simulink model "cw16"  (Simulink 7.0)
settings: Solver=ode4  StartTime=0.0  StopTime=10.0  FixedStep=0.01  RelTol=1e-3
values from neighbouring files (symbols this model uses):
  Beta_rate = 3*(pi/180)    (= 0.0523598775598)    [cw16set.m]
  g = 9.80665    [cw16set.m]
  gainfx = 1    [cw16set.m]
  gainfxtilt = 1    [cw16set.m]
  gainfy = 1    [cw16set.m]
  gainfytilt = 1    [cw16set.m]
  gainfz = 1    [cw16set.m]
  gainp = 1    [cw16set.m]
  gainq = 1    [cw16set.m]
  gainr = 1    [cw16set.m]
  HPomegabphi = 0.0    (= 0)    [cw16set.m]
  HPomegabpsi = 0.0    (= 0)    [cw16set.m]
  HPomegabtheta = 0.0    (= 0)    [cw16set.m]
  HPomegabx = 0.0    (= 0)    [cw16set.m]
  HPomegaby = 0.0    (= 0)    [cw16set.m]
  HPomegabz = 0.2    [cw16set.m]
  HPomeganphi = 1.0    (= 1)    [cw16set.m]
  HPomeganpsi = 1.0    (= 1)    [cw16set.m]
  HPomegantheta = 0.8    [cw16set.m]
  HPomeganx = 0.8    [cw16set.m]
  HPomegany = 1.0    (= 1)    [cw16set.m]
  HPomeganz = 1.0    (= 1)    [cw16set.m]
  HPzetaphi = 1.0    (= 1)    [cw16set.m]
  HPzetapsi = 1.0    (= 1)    [cw16set.m]
  HPzetatheta = 1.0    (= 1)    [cw16set.m]
  HPzetax = 1.0    (= 1)    [cw16set.m]
  HPzetay = 1.0    (= 1)    [cw16set.m]
  HPzetaz = 1.0    (= 1)    [cw16set.m]
  kf = [kfx 0 0; 0 kfy 0; 0 0 kfz]    [cw16set.m]
  Kfeedbackeuler = 0.2    [cw16set.m]
  Kfeedbackeulerrate = 0.5    [cw16set.m]
  Kfeedbackx = 0.5    [cw16set.m]
  Kfeedbackxd = 0.1    [cw16set.m]
  Ktilteuler = 0.2    [cw16set.m]
  Ktilteulerrate = 0.5    [cw16set.m]
  Ktiltrate = 5.0    (= 5)    [cw16set.m]
  kw = [kwp 0 0; 0 kwq 0; 0 0 kwr]    [cw16set.m]
  LPomeganx = 2.0    (= 2)    [cw16set.m]
  LPomegany = 2.0    (= 2)    [cw16set.m]
  LPzetax = 1.0    (= 1)    [cw16set.m]
  LPzetay = 1.0    (= 1)    [cw16set.m]
  LZDERPUGP = 1.2075    [cw16set.m]
  tiltcoordinationmethod = 1    [cw16set.m]
  xref_ac = 0.0    (= 0)    [cw16set.m]
  xref_filt = 0.0    (= 0)    [cw16set.m]
  yref_ac = 0.0    (= 0)    [cw16set.m]
  yref_filt = 0.0    (= 0)    [cw16set.m]
  zref_ac = -1.2075    [cw16set.m]
  zref_filt = 0.0    (= 0)    [cw16set.m]
libraries: simulink x4
(part 1 of 2)
settings Model: Creator=ostroosma  LastModifiedBy=ostroosma  ModifiedHistory=1.96: changed frequency of differentiating filters in tilt coordination from 12.5 to 50 rad/s  ParamWorkspaceSource=ReferencedWorkspace  ExtModeTrigMode=oneshot  ExtModeArmWhenConnect=off  TunableVars=Beta_rate,HPomegabphi,HPomegabpsi,HPomegabtheta,HPomegabx,HPomegaby,HPomegabz,HPomeganphi,HPomeganpsi,HPomegantheta,HPomeganx,HPomegany,HPomeganz,HPzetaphi,HPzetapsi,HPzetatheta,HPzetax,HPzetay,HPzetaz,Ktilteuler,Ktilteulerrate,Ktiltrate,LPomeganx,LPomegany,LPzetax,LPzetay,gainfx,gainfxtilt,gainfy,gainfytilt,gainfz,gainp,gainq,gainr,kf,kw,tiltcoordinationmethod,xref_ac,xref_filt,yref_ac,yref_filt,zref_ac,zref_filt  TunableVarsStorageClass=Auto,Auto,Auto,Auto,Auto,Auto,Auto,Auto,Auto,Auto,Auto,Auto,Auto,Auto,Auto,Auto,Auto,Auto,Auto,Auto,Auto,Auto,Auto,Auto,Auto,Auto,Auto,Auto,Auto,Auto,Auto,Auto,Auto,Auto,Auto,Auto,Auto,Auto,Auto,Auto,Auto,Auto,Auto  TunableVarsTypeQualifier=,,,,,,,,,,,,,,,,,,,,,,,,,,,,,,,,,,,,,,,,,,
settings DataIOCC: LimitDataPoints=off  SaveOutput=off  SignalLogging=off  SaveTime=off  SignalLoggingName=sigsOut
settings OptimizationCC: BooleanDataType=off  InlineParams=on
settings DebuggingCC: SaveWithParameterizedLinksMsg=none  SignalResolutionControl=TryResolveAllWithWarning  SolverPrmCheckMsg=none  MultiTaskDSMMsg=warning  MultiTaskCondExecSysMsg=none  FcnCallInpInsideContextMsg=Enable All  StrictBusMsg=ErrorLevel1
settings HardwareCC: TargetEndianess=LittleEndian  TargetHWDeviceType=MATLAB Host
settings RTWCC: SystemTargetFile=grt_malloc.tlc  GenCodeOnly=on  GenerateMakefile=off  TemplateMakefile=grt_malloc_default_tmf  Description=Generic Real-Time Target with dynamic memory allocation  ProcessScript=grt_malloc_make_rtw_hook  IncludeERTFirstTime=on
settings GRTTargetCC: ExtModeMexFile=noextcomm

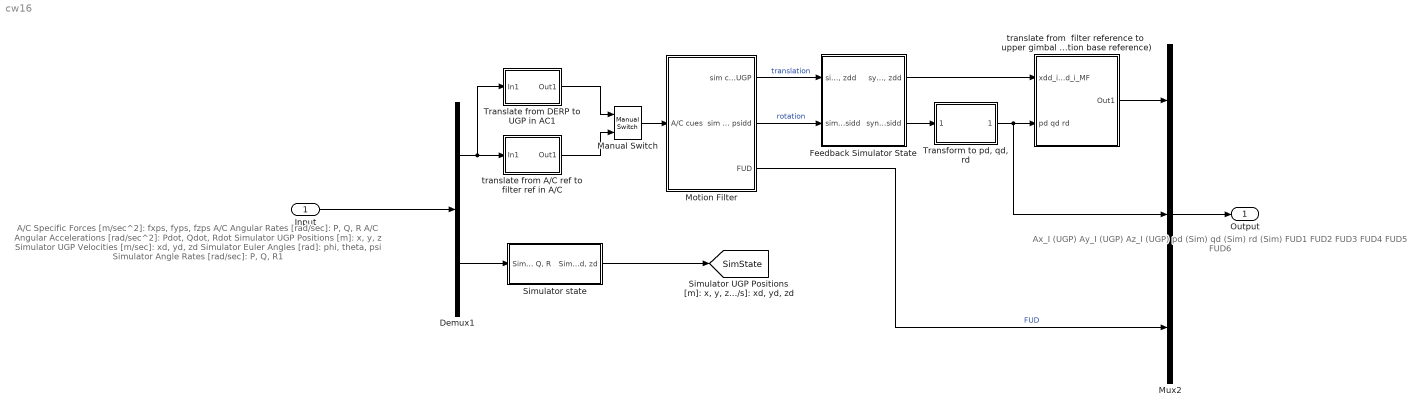
== system cw16 ==
  note: Ax_I (UGP)
      | Ay_I (UGP)
      | Az_I (UGP)
      | pd (Sim)
      | qd (Sim)
      | rd (Sim)
      | FUD1
      | FUD2
      | FUD3
      | FUD4
      | FUD5
      | FUD6
  note: A/C Specific Forces [m/sec^2]: fxps, fyps, fzps
      | A/C Angular Rates [rad/sec]: P, Q, R
      | A/C Angular Accelerations [rad/sec^2]: Pdot, Qdot, Rdot
      | Simulator UGP Positions [m]: x, y, z
      | Simulator UGP Velocities [m/sec]: xd, yd, zd
      | Simulator Euler Angles [rad]: phi, theta, psi
      | Simulator Angle Rates [rad/sec]: P, Q, R1
  Input : Inport
  Demux1 : Demux  Outputs=[9;12]
  Feedback Simulator State : Subsystem
  Manual Switch : simulink/Signal Routing/Manual Switch  SystemSampleTime=-1  sw=0  action=0  varsize=off
  Motion Filter : Subsystem
  Mux2 : Mux  Inputs=3
  Simulator state : Subsystem
  "Transform to pd, qd, rd" : Subsystem
  Translate from DERP to UGP in AC1 : Subsystem
  translate from  filter reference to  upper gimbal point  (motion base reference) : Subsystem
  translate from A/C ref to filter ref in A/C : Subsystem
  Output : Outport
  tag scope: SimState=global
  wires:
  Input/1 -> Demux1/1
  Motion Filter/1(sim commands: xdd_i_UGP ydd_i_UGP zdd_i_UGP) -> Feedback Simulator State/1("sim commands xdd, ydd, zdd")  "translation"
  Motion Filter/2(sim commands: phidd thetadd psidd) -> Feedback Simulator State/2(sim commands phidd thetadd psidd)  "rotation"
  Feedback Simulator State/2("synchronizing phidd, thetadd, psidd") -> "Transform to pd, qd, rd"/1(commands 1: phidd 2: thetadd 3: psidd)
  "Transform to pd, qd, rd"/1(pd qd rd) -> Mux2/2, translate from  filter reference to  upper gimbal point  (motion base reference)/2(pd qd rd)
  Mux2/1 -> Output/1
  Motion Filter/3(FUD) -> Mux2/3  "FUD"
  Demux1/1 -> Translate from DERP to UGP in AC1/1(In1), translate from A/C ref to filter ref in A/C/1(In1)
  Translate from DERP to UGP in AC1/1(Out1) -> Manual Switch/1
  translate from A/C ref to filter ref in A/C/1(Out1) -> Manual Switch/2
  Manual Switch/1 -> Motion Filter/1(A/C cues)
  Feedback Simulator State/1("synchronizing xdd, ydd, zdd") -> translate from  filter reference to  upper gimbal point  (motion base reference)/1(xdd_i_MF ydd_i_MF zdd_i_MF)
  translate from  filter reference to  upper gimbal point  (motion base reference)/1(Out1) -> Mux2/1
  Simulator state/1("Simulator UGP Positions [m]: x, y, z Simulator UGP Velocities [m/sec]: xd, yd, zd Simulator Euler Angles [rad]: phi, theta, psi Simulator Angle Rates [rad/sec]: P, Q, R Simulator Euler Angle Rates [rad/s]: phid, thetad, psid Simulator Filter Positions [m]: x, y, z Simulator Filter Velocities [m/s]: xd, yd, zd") -> [SimState]
  Demux1/2 -> Simulator state/1("Simulator UGP Positions [m]: x, y, z Simulator UGP Velocities [m/sec]: xd, yd, zd Simulator Euler Angles [rad]: phi, theta, psi Simulator Angle Rates [rad/sec]: P, Q, R")

== system cw16/Feedback Simulator State ==
  "sim commands xdd, ydd, zdd" : Inport
  sim commands phidd thetadd psidd : Inport  Port=2
  Demux : Demux  Outputs=[6;6]
  Euler angle and angular rate Feedback : Subsystem
  Position Velocity Feedback : Subsystem
  Sum4 : Sum  Inputs=|++  SaturateOnIntegerOverflow=on  InputSameDT=on
  Sum5 : Sum  Inputs=++|  SaturateOnIntegerOverflow=on  InputSameDT=on
  "x, y, z xd, yd, zd phi, theta, psi phid, thetad, psid" : Selector  InputPortWidth=21  IndexOptions=Index vector (dialog)  Indices=[16 17 18 19 20 21 7 8 9 13 14 15]  OutputSizes=1
  "synchronizing xdd, ydd, zdd" : Outport
  "synchronizing phidd, thetadd, psidd" : Outport  Port=2
  wires:
  sim commands phidd thetadd psidd/1 -> Sum4/1, Euler angle and angular rate Feedback/1("Simulator desired angular accelerations ")
  "sim commands xdd, ydd, zdd"/1 -> Sum5/2, Position Velocity Feedback/2("Simulator desired accelerations ")
  Euler angle and angular rate Feedback/1(feedback angular acceleration) -> Sum4/2
  Sum5/1 -> "synchronizing xdd, ydd, zdd"/1
  Sum4/1 -> "synchronizing phidd, thetadd, psidd"/1
  "x, y, z xd, yd, zd phi, theta, psi phid, thetad, psid"/1 -> Demux/1
  Demux/2 -> Euler angle and angular rate Feedback/2(feedback simulator state)
  Demux/1 -> Position Velocity Feedback/1(feedback simulator state)
  Position Velocity Feedback/1(feedback acceleration) -> Sum5/1
  [SimState] -> "x, y, z xd, yd, zd phi, theta, psi phid, thetad, psid"/1

== system cw16/Motion Filter ==
  A/C cues : Inport
  Demux1 : Demux  Outputs=[3;6]
  High Pass Channel Angular Accelerations : Subsystem
  High Pass Channel Specific Forces : Subsystem
  Low Pass Channel Specific Forces : Subsystem
  Sum1 : Sum  Inputs=++|  SaturateOnIntegerOverflow=on  InputSameDT=on
  f-scale : Subsystem
  w-scale : Subsystem
  sim commands: xdd_i_UGP ydd_i_UGP zdd_i_UGP : Outport
  sim commands: phidd thetadd psidd : Outport  Port=2
  FUD : Outport  Port=3
  wires:
  f-scale/1(scaled A/C specific force UGP) -> Low Pass Channel Specific Forces/1(scaled AC specific forces @ UGP), High Pass Channel Specific Forces/1(In1)
  Low Pass Channel Specific Forces/1(phidd LP thetadd LP psidd LP) -> Sum1/1
  Demux1/1 -> f-scale/1(A/C specific forces UGP)
  High Pass Channel Specific Forces/1(Out1) -> sim commands: xdd_i_UGP ydd_i_UGP zdd_i_UGP/1
  A/C cues/1 -> Demux1/1
  Sum1/1 -> sim commands: phidd thetadd psidd/1
  High Pass Channel Angular Accelerations/1(Out1) -> Sum1/2
  Demux1/2 -> w-scale/1(In1)
  w-scale/1(Out1) -> High Pass Channel Angular Accelerations/1(In1)
  Low Pass Channel Specific Forces/2(FUD) -> FUD/1

== system cw16/Simulator state ==
  "Simulator UGP Positions [m]: x, y, z Simulator UGP Velocities [m/sec]: xd, yd, zd Simulator Euler Angles [rad]: phi, theta, psi Simulator Angle Rates [rad/sec]: P, Q, R" : Inport
  Demux : Demux  Outputs=[6 6]
  Demux1 : Demux  Outputs=[3 3]
  Mux : Mux  Inputs=[6 6 3 3 3]
  "calculate position and velocity in filter reference point, for state feedback inside filter" : Stateflow chart  TreatAsAtomicUnit=on
  phi_s theta_s psi_s p_s q_s r_s : Selector  InputPortWidth=12  IndexOptions=Index vector (dialog)  Indices=[7 8 9 10 11 12]  OutputSizes=1
  reference points : Subsystem
  transformation to Euler angle rates : Subsystem
  "Simulator UGP Positions [m]: x, y, z Simulator UGP Velocities [m/sec]: xd, yd, zd Simulator Euler Angles [rad]: phi, theta, psi Simulator Angle Rates [rad/sec]: P, Q, R Simulator Euler Angle Rates [rad/s]: phid, thetad, psid Simulator Filter Positions [m]: x, y, z Simulator Filter Velocities [m/s]: xd, yd, zd" : Outport
  wires:
  "Simulator UGP Positions [m]: x, y, z Simulator UGP Velocities [m/sec]: xd, yd, zd Simulator Euler Angles [rad]: phi, theta, psi Simulator Angle Rates [rad/sec]: P, Q, R"/1 -> phi_s theta_s psi_s p_s q_s r_s/1, Demux/1
  Mux/1 -> "Simulator UGP Positions [m]: x, y, z Simulator UGP Velocities [m/sec]: xd, yd, zd Simulator Euler Angles [rad]: phi, theta, psi Simulator Angle Rates [rad/sec]: P, Q, R Simulator Euler Angle Rates [rad/s]: phid, thetad, psid Simulator Filter Positions [m]: x, y, z Simulator Filter Velocities [m/s]: xd, yd, zd"/1
  Demux/1 -> Demux1/1, Mux/1
  Demux/2 -> Mux/2, transformation to Euler angle rates/1("phi theta psi p q r ")
  transformation to Euler angle rates/1(phidot thetadot psidot) -> Mux/3
  reference points/1(Out1) -> "calculate position and velocity in filter reference point, for state feedback inside filter"/4(refpos)
  phi_s theta_s psi_s p_s q_s r_s/1 -> "calculate position and velocity in filter reference point, for state feedback inside filter"/3(attsim)
  Demux1/2 -> "calculate position and velocity in filter reference point, for state feedback inside filter"/2(xd_ugp)
  Demux1/1 -> "calculate position and velocity in filter reference point, for state feedback inside filter"/1(x_ugp)
  "calculate position and velocity in filter reference point, for state feedback inside filter"/1(x_filt) -> Mux/4
  "calculate position and velocity in filter reference point, for state feedback inside filter"/2(xd_filt) -> Mux/5

== system cw16/Transform to pd, qd, rd ==
  note: differentiated formula 2.14 from UTIAS
  note: WHY, it's in SimState already?
  commands 1: phidd 2: thetadd 3: psidd : Inport
  7: phi 8: theta 9: psi 10: phid 11: thetad 12: psid : Selector  InputPortWidth=21  IndexOptions=Index vector (dialog)  Indices=[7 8 9 13 14 15]  OutputSizes=1
  Integrate to  4: phid 5: thetad 6: psid : Subsystem
  Mux : Mux  Inputs=3
  Mux1 : Mux  Inputs=3
  pd : Fcn  Expr=-cos(u[8])*u[11]*u[6]+u[1]-sin(u[8])*u[3]
  qd : Fcn  Expr=-sin(u[7])*u[10]*u[5]+(cos(u[8])*cos(u[7])*u[10]-sin(u[8])*u[11]*sin(u[7]))*u[6]+cos(u[7])*u[2]+cos(u[8])*sin(u[7])*u[3]
  rd : Fcn  Expr=-cos(u[7])*u[10]*u[5]-(sin(u[8])*u[11]*cos(u[7])+cos(u[8])*sin(u[7])*u[10])*u[6]-sin(u[7])*u[2]+cos(u[8])*cos(u[7])*u[3]
  pd qd rd : Outport
  wires:
  commands 1: phidd 2: thetadd 3: psidd/1 -> Integrate to  4: phid 5: thetad 6: psid/1(In1), Mux/1
  Integrate to  4: phid 5: thetad 6: psid/1(Out1) -> Mux/2
  Mux/1 -> pd/1, qd/1, rd/1
  qd/1 -> Mux1/2
  rd/1 -> Mux1/3
  pd/1 -> Mux1/1
  Mux1/1 -> pd qd rd/1
  [SimState] -> 7: phi 8: theta 9: psi 10: phid 11: thetad 12: psid/1
  7: phi 8: theta 9: psi 10: phid 11: thetad 12: psid/1 -> Mux/3

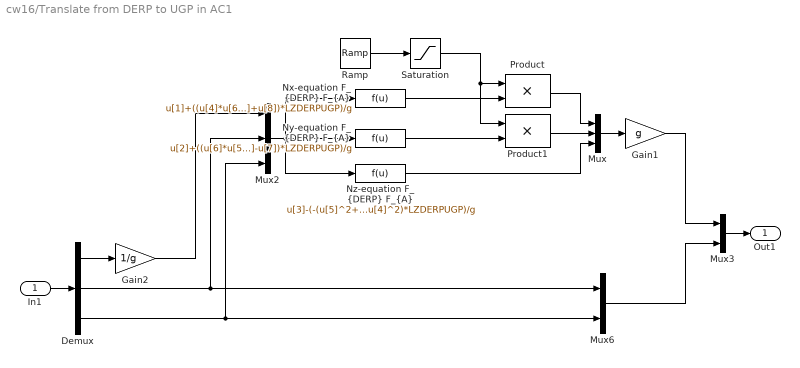
== system cw16/Translate from DERP to UGP in AC1 ==
  In1 : Inport
  Demux : Demux  Outputs=[3;3;3]
  Gain1 : Gain  Gain=g  SaturateOnIntegerOverflow=on
  Gain2 : Gain  Gain=1/g  SaturateOnIntegerOverflow=on
  Mux : Mux  Inputs=3
  Mux2 : Mux  Inputs=3
  Mux3 : Mux  Inputs=2
  Mux6 : Mux  Inputs=2
  "Nx-equation F_{DERP} F_{A}" : Fcn  Expr=u[1]+((u[4]*u[6]+u[8])*LZDERPUGP)/g
  "Ny-equation F_{DERP} F_{A}" : Fcn  Expr=u[2]+((u[6]*u[5]-u[7])*LZDERPUGP)/g
  "Nz-equation F_{DERP} F_{A}" : Fcn  Expr=u[3]-(-(u[5]^2+u[4]^2)*LZDERPUGP)/g
  Product : Product  SaturateOnIntegerOverflow=on  InputSameDT=on
  Product1 : Product  SaturateOnIntegerOverflow=on  InputSameDT=on
  Ramp : simulink/Sources/Ramp  SystemSampleTime=-1  slope=0.2  start=0  X0=0
  Saturation : Saturate  UpperLimit=1  LowerLimit=0
  Out1 : Outport
  wires:
  Mux2/1 -> "Ny-equation F_{DERP} F_{A}"/1, "Nx-equation F_{DERP} F_{A}"/1, "Nz-equation F_{DERP} F_{A}"/1
  Ramp/1 -> Saturation/1
  Mux/1 -> Gain1/1
  Product/1 -> Mux/1
  "Nx-equation F_{DERP} F_{A}"/1 -> Product/2
  Product1/1 -> Mux/2
  "Ny-equation F_{DERP} F_{A}"/1 -> Product1/2
  Saturation/1 -> Product/1, Product1/1
  Gain1/1 -> Mux3/1
  Mux6/1 -> Mux3/2
  Mux3/1 -> Out1/1
  In1/1 -> Demux/1
  Demux/3 -> Mux2/3, Mux6/2
  Demux/2 -> Mux2/2, Mux6/1
  Demux/1 -> Gain2/1
  Gain2/1 -> Mux2/1
  "Nz-equation F_{DERP} F_{A}"/1 -> Mux/3

== system cw16/translate from  filter reference to  upper gimbal point  (motion base reference) ==
  xdd_i_MF ydd_i_MF zdd_i_MF : Inport  PortDimensions=3
  pd qd rd : Inport  Port=2
  move inertial acceleration setpoints in MF reference point to UGP reference point : Stateflow chart  TreatAsAtomicUnit=on
  phi_s theta_s psi_s p_s q_s r_s : Selector  InputPortWidth=21  IndexOptions=Index vector (dialog)  Indices=[7 8 9 10 11 12]  OutputSizes=1
  reference points : Subsystem
  Out1 : Outport
  wires:
  xdd_i_MF ydd_i_MF zdd_i_MF/1 -> move inertial acceleration setpoints in MF reference point to UGP reference point/1(xdd_i_mf)
  reference points/1(Out1) -> move inertial acceleration setpoints in MF reference point to UGP reference point/4(refpos)
  move inertial acceleration setpoints in MF reference point to UGP reference point/1(xdd_i_ugp) -> Out1/1
  pd qd rd/1 -> move inertial acceleration setpoints in MF reference point to UGP reference point/2(wd_mf)
  [SimState] -> phi_s theta_s psi_s p_s q_s r_s/1
  phi_s theta_s psi_s p_s q_s r_s/1 -> move inertial acceleration setpoints in MF reference point to UGP reference point/3(attsim)

== system cw16/translate from A/C ref to filter ref in A/C ==
  note: fade in fx/fy
  In1 : Inport
  Demux : Demux  Outputs=[2 7]
  Embedded MATLAB Function : Stateflow chart  TreatAsAtomicUnit=on
  Mux : Mux  Inputs=[2 7]
  Product : Product  SaturateOnIntegerOverflow=on  InputSameDT=on
  Ramp : simulink/Sources/Ramp  SystemSampleTime=-1  slope=0.2  start=0  X0=0
  Saturation : Saturate  UpperLimit=1  LowerLimit=0
  reference points : Subsystem
  Out1 : Outport
  wires:
  Embedded MATLAB Function/1(y) -> Out1/1
  reference points/1(Out1) -> Embedded MATLAB Function/2(refpos)
  Ramp/1 -> Saturation/1
  Saturation/1 -> Product/1
  In1/1 -> Demux/1
  Demux/1 -> Product/2
  Product/1 -> Mux/1
  Demux/2 -> Mux/2
  Mux/1 -> Embedded MATLAB Function/1(u)

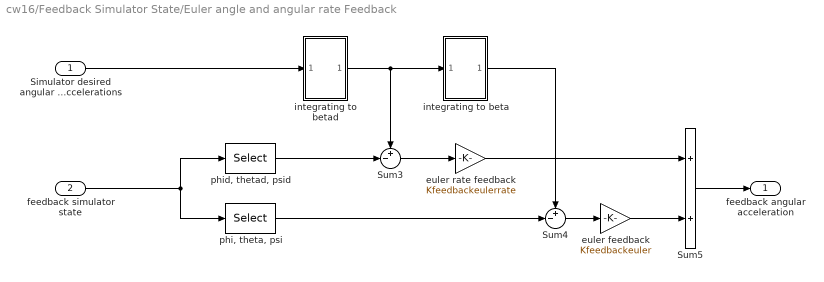
== system cw16/Feedback Simulator State/Euler angle and angular rate Feedback ==
  "Simulator desired angular accelerations " : Inport
  feedback simulator state : Inport  Port=2
  Sum3 : Sum  Inputs=+-|  SaturateOnIntegerOverflow=on  InputSameDT=on
  Sum4 : Sum  Inputs=+-|  SaturateOnIntegerOverflow=on  InputSameDT=on
  Sum5 : Sum  SaturateOnIntegerOverflow=on  InputSameDT=on
  euler feedback : Gain  Gain=Kfeedbackeuler  SaturateOnIntegerOverflow=on
  euler rate feedback : Gain  Gain=Kfeedbackeulerrate  SaturateOnIntegerOverflow=on
  integrating to beta : Subsystem
  integrating to betad : Subsystem
  "phi, theta, psi" : Selector  InputPortWidth=6  IndexOptions=Index vector (dialog)  Indices=[1 2 3]  OutputSizes=1
  "phid, thetad, psid" : Selector  InputPortWidth=6  IndexOptions=Index vector (dialog)  Indices=[4 5 6]  OutputSizes=1
  feedback angular acceleration : Outport
  wires:
  "Simulator desired angular accelerations "/1 -> integrating to betad/1(In1)
  integrating to betad/1(Out1) -> integrating to beta/1(In1), Sum3/1
  Sum3/1 -> euler rate feedback/1
  feedback simulator state/1 -> "phi, theta, psi"/1, "phid, thetad, psid"/1
  integrating to beta/1(Out1) -> Sum4/1
  Sum4/1 -> euler feedback/1
  euler feedback/1 -> Sum5/2
  euler rate feedback/1 -> Sum5/1
  Sum5/1 -> feedback angular acceleration/1
  "phi, theta, psi"/1 -> Sum4/2
  "phid, thetad, psid"/1 -> Sum3/2

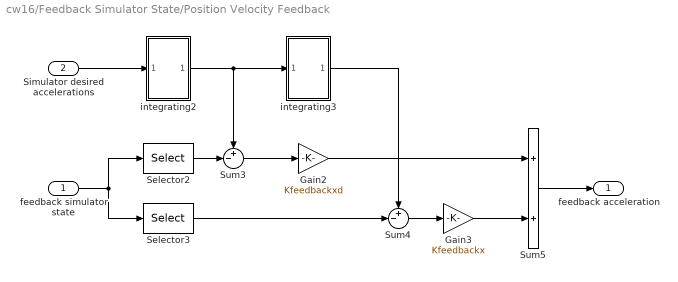
== system cw16/Feedback Simulator State/Position Velocity Feedback ==
  feedback simulator state : Inport
  "Simulator desired accelerations " : Inport  Port=2
  Gain2 : Gain  Gain=Kfeedbackxd  SaturateOnIntegerOverflow=on
  Gain3 : Gain  Gain=Kfeedbackx  SaturateOnIntegerOverflow=on
  Selector2 : Selector  InputPortWidth=6  IndexOptions=Index vector (dialog)  Indices=[4 5 6]  OutputSizes=1
  Selector3 : Selector  InputPortWidth=6  IndexOptions=Index vector (dialog)  Indices=[1 2 3]  OutputSizes=1
  Sum3 : Sum  Inputs=+-|  SaturateOnIntegerOverflow=on  InputSameDT=on
  Sum4 : Sum  Inputs=+-|  SaturateOnIntegerOverflow=on  InputSameDT=on
  Sum5 : Sum  SaturateOnIntegerOverflow=on  InputSameDT=on
  integrating2 : Subsystem
  integrating3 : Subsystem
  feedback acceleration : Outport
  wires:
  "Simulator desired accelerations "/1 -> integrating2/1(In1)
  Selector2/1 -> Sum3/2
  integrating2/1(Out1) -> integrating3/1(In1), Sum3/1
  Sum3/1 -> Gain2/1
  feedback simulator state/1 -> Selector2/1, Selector3/1
  Selector3/1 -> Sum4/2
  integrating3/1(Out1) -> Sum4/1
  Sum4/1 -> Gain3/1
  Gain3/1 -> Sum5/2
  Gain2/1 -> Sum5/1
  Sum5/1 -> feedback acceleration/1

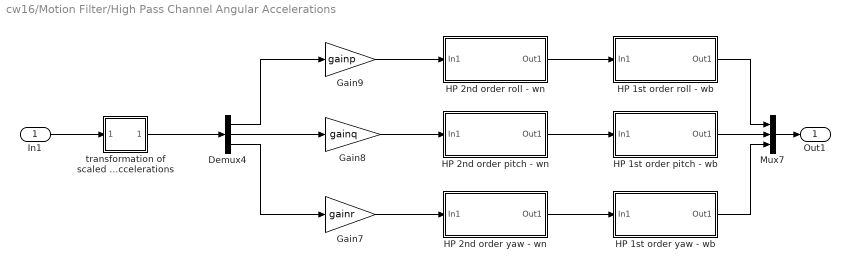
== system cw16/Motion Filter/High Pass Channel Angular Accelerations ==
  In1 : Inport
  Demux4 : Demux  Outputs=3
  Gain7 : Gain  Gain=gainr  SaturateOnIntegerOverflow=on
  Gain8 : Gain  Gain=gainq  SaturateOnIntegerOverflow=on
  Gain9 : Gain  Gain=gainp  SaturateOnIntegerOverflow=on
  HP 1st order pitch - wb : Subsystem
  HP 1st order roll - wb : Subsystem
  HP 1st order yaw - wb : Subsystem
  HP 2nd order pitch - wn : Subsystem
  HP 2nd order roll - wn : Subsystem
  HP 2nd order yaw - wn : Subsystem
  Mux7 : Mux  Inputs=3
  transformation of scaled A/C rotations to sim Euler angle accelerations : Subsystem
  Out1 : Outport
  wires:
  Gain7/1 -> HP 2nd order yaw - wn/1(In1)
  Gain8/1 -> HP 2nd order pitch - wn/1(In1)
  Gain9/1 -> HP 2nd order roll - wn/1(In1)
  Demux4/1 -> Gain9/1
  Demux4/3 -> Gain7/1
  In1/1 -> transformation of scaled A/C rotations to sim Euler angle accelerations/1(1: p (A/C) 2: q (A/C) 3: r (A/C) 4: pd (A/C) 5: qd (A/C) 6: rd (A/C))
  Demux4/2 -> Gain8/1
  transformation of scaled A/C rotations to sim Euler angle accelerations/1(phidd thetadd psidd) -> Demux4/1
  Mux7/1 -> Out1/1
  HP 1st order roll - wb/1(Out1) -> Mux7/1
  HP 1st order pitch - wb/1(Out1) -> Mux7/2
  HP 1st order yaw - wb/1(Out1) -> Mux7/3
  HP 2nd order roll - wn/1(Out1) -> HP 1st order roll - wb/1(In1)
  HP 2nd order pitch - wn/1(Out1) -> HP 1st order pitch - wb/1(In1)
  HP 2nd order yaw - wn/1(Out1) -> HP 1st order yaw - wb/1(In1)

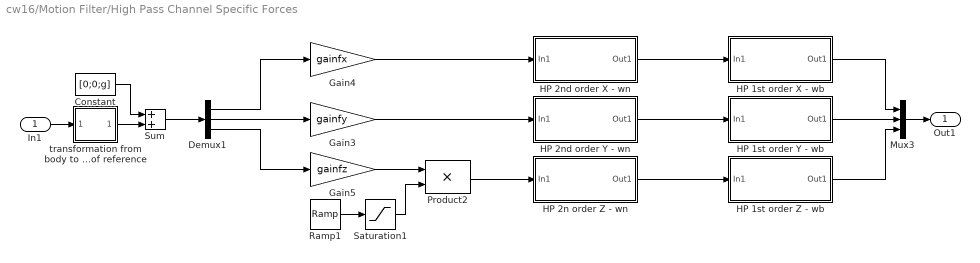
== system cw16/Motion Filter/High Pass Channel Specific Forces ==
  In1 : Inport
  Constant : Constant  Value=[0;0;g]
  Demux1 : Demux  Outputs=3
  Gain3 : Gain  Gain=gainfy  SaturateOnIntegerOverflow=on
  Gain4 : Gain  Gain=gainfx  SaturateOnIntegerOverflow=on
  Gain5 : Gain  Gain=gainfz  SaturateOnIntegerOverflow=on
  HP 1st order X - wb : Subsystem
  HP 1st order Y - wb : Subsystem
  HP 1st order Z - wb : Subsystem
  HP 2n order Z - wn : Subsystem
  HP 2nd order X - wn : Subsystem
  HP 2nd order Y - wn : Subsystem
  Mux3 : Mux  Inputs=3
  Product2 : Product  SaturateOnIntegerOverflow=on  InputSameDT=on
  Ramp1 : simulink/Sources/Ramp  SystemSampleTime=-1  slope=0.2  start=0  X0=0
  Saturation1 : Saturate  UpperLimit=1  LowerLimit=0
  Sum : Sum  SaturateOnIntegerOverflow=on  InputSameDT=on
  transformation from body to inertial frame of reference : Subsystem
  Out1 : Outport
  wires:
  transformation from body to inertial frame of reference/1(fxI fyI fzI) -> Sum/2
  Constant/1 -> Sum/1
  Sum/1 -> Demux1/1
  Demux1/2 -> Gain3/1
  Demux1/1 -> Gain4/1
  Demux1/3 -> Gain5/1
  Gain3/1 -> HP 2nd order Y - wn/1(In1)
  HP 2nd order Y - wn/1(Out1) -> HP 1st order Y - wb/1(In1)
  HP 2nd order X - wn/1(Out1) -> HP 1st order X - wb/1(In1)
  HP 2n order Z - wn/1(Out1) -> HP 1st order Z - wb/1(In1)
  HP 1st order Y - wb/1(Out1) -> Mux3/2
  Product2/1 -> HP 2n order Z - wn/1(In1)
  Gain5/1 -> Product2/1
  Saturation1/1 -> Product2/2
  Ramp1/1 -> Saturation1/1
  HP 1st order Z - wb/1(Out1) -> Mux3/3
  Mux3/1 -> Out1/1
  In1/1 -> transformation from body to inertial frame of reference/1(fxS fyS fzS)
  HP 1st order X - wb/1(Out1) -> Mux3/1
  Gain4/1 -> HP 2nd order X - wn/1(In1)

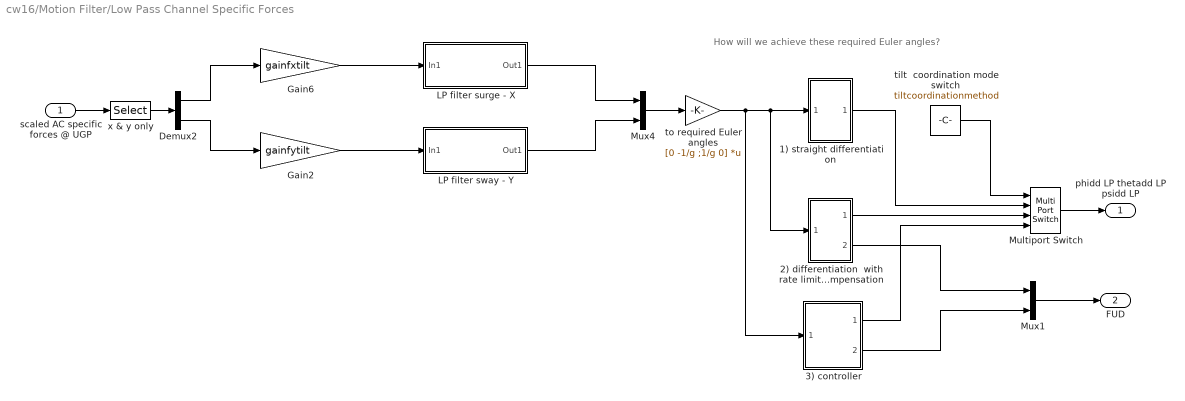
== system cw16/Motion Filter/Low Pass Channel Specific Forces ==
  note: How will we achieve
      | these required Euler angles?
  scaled AC specific forces @ UGP : Inport
  1) straight differentiation : Subsystem
  2) differentiation  with rate limit  compensation : Subsystem
  3) controller : Subsystem
  Demux2 : Demux  Outputs=2
  Gain2 : Gain  Gain=gainfytilt  SaturateOnIntegerOverflow=on
  Gain6 : Gain  Gain=gainfxtilt  SaturateOnIntegerOverflow=on
  "LP filter surge - X " : Subsystem
  "LP filter sway - Y " : Subsystem
  Multiport Switch : MultiPortSwitch  Inputs=3  SaturateOnIntegerOverflow=on
  Mux1 : Mux  Inputs=[3 3]
  Mux4 : Mux  Inputs=2
  tilt  coordination mode switch : Constant  Value=tiltcoordinationmethod
  to required Euler angles : Gain  Gain=[0 -1/g ;1/g 0]  Multiplication=Matrix(K*u)  SaturateOnIntegerOverflow=on
  x & y only : Selector  InputPortWidth=3  IndexOptions=Index vector (dialog)  Indices=[1 2]  OutputSizes=1
  phidd LP thetadd LP psidd LP : Outport
  FUD : Outport  Port=2
  wires:
  scaled AC specific forces @ UGP/1 -> x & y only/1
  x & y only/1 -> Demux2/1
  Gain2/1 -> "LP filter sway - Y "/1(In1)
  Gain6/1 -> "LP filter surge - X "/1(In1)
  "LP filter sway - Y "/1(Out1) -> Mux4/2
  "LP filter surge - X "/1(Out1) -> Mux4/1
  Mux4/1 -> to required Euler angles/1
  to required Euler angles/1 -> 3) controller/1(required Euler angles: phi theta), 1) straight differentiation/1(phi lp theta lp), 2) differentiation  with rate limit  compensation/1(phi lp theta lp)
  Demux2/2 -> Gain2/1
  Demux2/1 -> Gain6/1
  Multiport Switch/1 -> phidd LP thetadd LP psidd LP/1
  1) straight differentiation/1(phidd lp thetadd lp psidd lp) -> Multiport Switch/2
  3) controller/1(phidd lp thetadd lp psidd lp) -> Multiport Switch/4
  2) differentiation  with rate limit  compensation/1(phidd lp thetadd lp psidd lp) -> Multiport Switch/3
  tilt  coordination mode switch/1 -> Multiport Switch/1
  Mux1/1 -> FUD/1
  2) differentiation  with rate limit  compensation/2(theta req theta lim controller thetad) -> Mux1/1
  3) controller/2("theta req theta sim thetadd controller ") -> Mux1/2

== system cw16/Motion Filter/f-scale ==
  A/C specific forces UGP : Inport
  Constant : Constant  Value=[0;0;g]
  Sum1 : Sum  Inputs=++|  SaturateOnIntegerOverflow=on  InputSameDT=on
  Sum2 : Sum  Inputs=-+|  SaturateOnIntegerOverflow=on  InputSameDT=on
  kf : Gain  Gain=kf  Multiplication=Matrix(K*u)  SaturateOnIntegerOverflow=on
  scaled A/C specific force UGP : Outport
  wires:
  Sum1/1 -> kf/1
  kf/1 -> Sum2/2
  Constant/1 -> Sum1/1, Sum2/1
  A/C specific forces UGP/1 -> Sum1/2
  Sum2/1 -> scaled A/C specific force UGP/1

== system cw16/Motion Filter/w-scale ==
  In1 : Inport
  Demux : Demux  Outputs=[3;3]
  Matrix Gain : Gain  Gain=kw  Multiplication=Matrix(K*u)  SaturateOnIntegerOverflow=on
  Matrix Gain1 : Gain  Gain=kw  Multiplication=Matrix(K*u)  SaturateOnIntegerOverflow=on
  Mux : Mux  Inputs=2
  Out1 : Outport
  wires:
  In1/1 -> Demux/1
  Mux/1 -> Out1/1
  Matrix Gain1/1 -> Mux/2
  Matrix Gain/1 -> Mux/1
  Demux/2 -> Matrix Gain1/1
  Demux/1 -> Matrix Gain/1

== system cw16/Simulator state/reference points ==
  note: This is stupid, but
      | necessary to keep
      | them tunable !?
      | Replacing with single array constant
      | doesn't work in R2007b
  Mux : Mux  Inputs=6
  xref_ac : Constant  Value=xref_ac
  xref_filt : Constant  Value=xref_filt
  yref_ac : Constant  Value=yref_ac
  yref_filt : Constant  Value=yref_filt
  zref_ac : Constant  Value=zref_ac
  zref_filt : Constant  Value=zref_filt
  Out1 : Outport
  wires:
  xref_ac/1 -> Mux/1
  yref_ac/1 -> Mux/2
  zref_ac/1 -> Mux/3
  xref_filt/1 -> Mux/4
  yref_filt/1 -> Mux/5
  zref_filt/1 -> Mux/6
  Mux/1 -> Out1/1

== system cw16/Simulator state/transformation to Euler angle rates ==
  note: transformation to Euler angle rates by eqn 2.12 from UTIAS doc
  "phi theta psi p q r " : Inport
  Mux : Mux  Inputs=3
  phidot : Fcn  Expr=u[4]+(u[5]*sin(u[1])+u[6]*cos(u[1]))*tan(u[2])
  psidot : Fcn  Expr=(u[5]*sin(u[1])+u[6]*cos(u[1]))/cos(u[2])
  thetadot : Fcn  Expr=u[5]*cos(u[1])-u[6]*sin(u[1])
  phidot thetadot psidot : Outport
  wires:
  Mux/1 -> phidot thetadot psidot/1
  "phi theta psi p q r "/1 -> thetadot/1, phidot/1, psidot/1
  phidot/1 -> Mux/1
  thetadot/1 -> Mux/2
  psidot/1 -> Mux/3

== system cw16/Transform to pd, qd, rd/Integrate to  4: phid 5: thetad 6: psid ==
  In1 : Inport
  Demux : Demux  Outputs=3
  Mux : Mux  Inputs=3
  Transfer Fcn : TransferFcn  Denominator=[1 0]
  Transfer Fcn1 : TransferFcn  Denominator=[1 0]
  Transfer Fcn2 : TransferFcn  Denominator=[1 0]
  Out1 : Outport
  wires:
  Demux/2 -> Transfer Fcn1/1
  Demux/3 -> Transfer Fcn2/1
  In1/1 -> Demux/1
  Demux/1 -> Transfer Fcn/1
  Transfer Fcn2/1 -> Mux/3
  Transfer Fcn1/1 -> Mux/2
  Transfer Fcn/1 -> Mux/1
  Mux/1 -> Out1/1

== system cw16/translate from  filter reference to  upper gimbal point  (motion base reference)/reference points ==
  note: This is stupid, but
      | necessary to keep
      | them tunable !?
      | Replacing with single array constant
      | doesn't work in R2007b
  Mux : Mux  Inputs=6
  xref_ac : Constant  Value=xref_ac
  xref_filt : Constant  Value=xref_filt
  yref_ac : Constant  Value=yref_ac
  yref_filt : Constant  Value=yref_filt
  zref_ac : Constant  Value=zref_ac
  zref_filt : Constant  Value=zref_filt
  Out1 : Outport
  wires:
  xref_ac/1 -> Mux/1
  yref_ac/1 -> Mux/2
  zref_ac/1 -> Mux/3
  xref_filt/1 -> Mux/4
  yref_filt/1 -> Mux/5
  zref_filt/1 -> Mux/6
  Mux/1 -> Out1/1

== system cw16/translate from A/C ref to filter ref in A/C/reference points ==
  note: This is stupid, but
      | necessary to keep
      | them tunable !?
      | Replacing with single array constant
      | doesn't work in R2007b
  Mux : Mux  Inputs=6
  xref_ac : Constant  Value=xref_ac
  xref_filt : Constant  Value=xref_filt
  yref_ac : Constant  Value=yref_ac
  yref_filt : Constant  Value=yref_filt
  zref_ac : Constant  Value=zref_ac
  zref_filt : Constant  Value=zref_filt
  Out1 : Outport
  wires:
  xref_ac/1 -> Mux/1
  yref_ac/1 -> Mux/2
  zref_ac/1 -> Mux/3
  xref_filt/1 -> Mux/4
  yref_filt/1 -> Mux/5
  zref_filt/1 -> Mux/6
  Mux/1 -> Out1/1

== system cw16/Feedback Simulator State/Euler angle and angular rate Feedback/integrating to beta ==
  In1 : Inport
  Demux : Demux  Outputs=3
  Integrator : Integrator
  Integrator1 : Integrator
  Integrator2 : Integrator
  Mux : Mux  Inputs=3
  Out1 : Outport
  wires:
  Demux/2 -> Integrator1/1
  In1/1 -> Demux/1
  Demux/1 -> Integrator/1
  Demux/3 -> Integrator2/1
  Integrator1/1 -> Mux/2
  Integrator/1 -> Mux/1
  Integrator2/1 -> Mux/3
  Mux/1 -> Out1/1

== system cw16/Feedback Simulator State/Euler angle and angular rate Feedback/integrating to betad ==
  In1 : Inport
  Demux : Demux  Outputs=3
  Integrator : Integrator
  Integrator1 : Integrator
  Integrator2 : Integrator
  Mux : Mux  Inputs=3
  Out1 : Outport
  wires:
  Demux/2 -> Integrator1/1
  In1/1 -> Demux/1
  Demux/1 -> Integrator/1
  Demux/3 -> Integrator2/1
  Integrator1/1 -> Mux/2
  Integrator/1 -> Mux/1
  Integrator2/1 -> Mux/3
  Mux/1 -> Out1/1

== system cw16/Feedback Simulator State/Position Velocity Feedback/integrating2 ==
  In1 : Inport
  Demux : Demux  Outputs=3
  Integrator : Integrator
  Integrator1 : Integrator
  Integrator2 : Integrator
  Mux : Mux  Inputs=3
  Out1 : Outport
  wires:
  Demux/2 -> Integrator1/1
  In1/1 -> Demux/1
  Demux/3 -> Integrator2/1
  Integrator1/1 -> Mux/2
  Integrator2/1 -> Mux/3
  Mux/1 -> Out1/1
  Demux/1 -> Integrator/1
  Integrator/1 -> Mux/1

== system cw16/Feedback Simulator State/Position Velocity Feedback/integrating3 ==
  In1 : Inport
  Demux : Demux  Outputs=3
  Integrator : Integrator  InitialCondition=xref_filt
  Integrator1 : Integrator  InitialCondition=yref_filt
  Integrator2 : Integrator  InitialCondition=zref_filt
  Mux : Mux  Inputs=3
  Out1 : Outport
  wires:
  Demux/2 -> Integrator1/1
  In1/1 -> Demux/1
  Demux/1 -> Integrator/1
  Demux/3 -> Integrator2/1
  Integrator1/1 -> Mux/2
  Integrator/1 -> Mux/1
  Integrator2/1 -> Mux/3
  Mux/1 -> Out1/1

== system cw16/Motion Filter/High Pass Channel Angular Accelerations/HP 1st order pitch - wb ==
  In1 : Inport
  Gain1 : Gain  Orientation=left  Gain=HPomegabtheta  SaturateOnIntegerOverflow=on
  Integrator2 : Integrator  Orientation=left
  Sum : Sum  Inputs=|+-  SaturateOnIntegerOverflow=on
  Out1 : Outport
  wires:
  In1/1 -> Sum/1
  Sum/1 -> Out1/1, Integrator2/1
  Integrator2/1 -> Gain1/1
  Gain1/1 -> Sum/2

== system cw16/Motion Filter/High Pass Channel Angular Accelerations/HP 1st order roll - wb ==
  In1 : Inport
  Gain1 : Gain  Orientation=left  Gain=HPomegabphi  SaturateOnIntegerOverflow=on
  Integrator2 : Integrator  Orientation=left
  Sum : Sum  Inputs=|+-  SaturateOnIntegerOverflow=on
  Out1 : Outport
  wires:
  In1/1 -> Sum/1
  Sum/1 -> Out1/1, Integrator2/1
  Integrator2/1 -> Gain1/1
  Gain1/1 -> Sum/2

== system cw16/Motion Filter/High Pass Channel Angular Accelerations/HP 1st order yaw - wb ==
  In1 : Inport
  Gain1 : Gain  Orientation=left  Gain=HPomegabpsi  SaturateOnIntegerOverflow=on
  Integrator2 : Integrator  Orientation=left
  Sum : Sum  Inputs=|+-  SaturateOnIntegerOverflow=on
  Out1 : Outport
  wires:
  In1/1 -> Sum/1
  Sum/1 -> Out1/1, Integrator2/1
  Integrator2/1 -> Gain1/1
  Gain1/1 -> Sum/2

== system cw16/Motion Filter/High Pass Channel Angular Accelerations/HP 2nd order pitch - wn ==
  In1 : Inport
  Gain : Gain  Orientation=left  Gain=HPomegantheta  SaturateOnIntegerOverflow=on
  Gain1 : Gain  Orientation=left  Gain=HPomegantheta  SaturateOnIntegerOverflow=on
  Gain2 : Gain  Orientation=left  Gain=HPomegantheta  SaturateOnIntegerOverflow=on
  Gain3 : Gain  Orientation=left  Gain=HPzetatheta  SaturateOnIntegerOverflow=on
  Gain4 : Gain  Orientation=left  Gain=2  SaturateOnIntegerOverflow=on
  Integrator2 : Integrator  Orientation=left
  Integrator3 : Integrator  Orientation=left
  Integrator4 : Integrator  Orientation=left
  Sum : Sum  Inputs=|+-  SaturateOnIntegerOverflow=on
  Sum1 : Sum  Orientation=left  Inputs=|++  SaturateOnIntegerOverflow=on
  Out1 : Outport
  wires:
  Gain1/1 -> Sum1/1
  Integrator2/1 -> Gain/1
  Gain/1 -> Gain1/1
  Integrator4/1 -> Gain3/1
  Integrator3/1 -> Integrator2/1
  Gain4/1 -> Sum1/2
  Gain2/1 -> Gain4/1
  Gain3/1 -> Gain2/1
  Sum1/1 -> Sum/2
  Sum/1 -> Out1/1, Integrator4/1, Integrator3/1
  In1/1 -> Sum/1

== system cw16/Motion Filter/High Pass Channel Angular Accelerations/HP 2nd order roll - wn ==
  In1 : Inport
  Gain : Gain  Orientation=left  Gain=HPomeganphi  SaturateOnIntegerOverflow=on
  Gain1 : Gain  Orientation=left  Gain=HPomeganphi  SaturateOnIntegerOverflow=on
  Gain2 : Gain  Orientation=left  Gain=HPomeganphi  SaturateOnIntegerOverflow=on
  Gain3 : Gain  Orientation=left  Gain=HPzetaphi  SaturateOnIntegerOverflow=on
  Gain4 : Gain  Orientation=left  Gain=2  SaturateOnIntegerOverflow=on
  Integrator2 : Integrator  Orientation=left
  Integrator3 : Integrator  Orientation=left
  Integrator4 : Integrator  Orientation=left
  Sum : Sum  Inputs=|+-  SaturateOnIntegerOverflow=on
  Sum1 : Sum  Orientation=left  Inputs=|++  SaturateOnIntegerOverflow=on
  Out1 : Outport
  wires:
  In1/1 -> Sum/1
  Sum/1 -> Integrator3/1, Integrator4/1, Out1/1
  Sum1/1 -> Sum/2
  Gain3/1 -> Gain2/1
  Gain2/1 -> Gain4/1
  Gain4/1 -> Sum1/2
  Integrator3/1 -> Integrator2/1
  Integrator4/1 -> Gain3/1
  Gain/1 -> Gain1/1
  Integrator2/1 -> Gain/1
  Gain1/1 -> Sum1/1

== system cw16/Motion Filter/High Pass Channel Angular Accelerations/HP 2nd order yaw - wn ==
  In1 : Inport
  Gain : Gain  Orientation=left  Gain=HPomeganpsi  SaturateOnIntegerOverflow=on
  Gain1 : Gain  Orientation=left  Gain=HPomeganpsi  SaturateOnIntegerOverflow=on
  Gain2 : Gain  Orientation=left  Gain=HPomeganpsi  SaturateOnIntegerOverflow=on
  Gain3 : Gain  Orientation=left  Gain=HPzetapsi  SaturateOnIntegerOverflow=on
  Gain4 : Gain  Orientation=left  Gain=2  SaturateOnIntegerOverflow=on
  Integrator2 : Integrator  Orientation=left
  Integrator3 : Integrator  Orientation=left
  Integrator4 : Integrator  Orientation=left
  Sum : Sum  Inputs=|+-  SaturateOnIntegerOverflow=on
  Sum1 : Sum  Orientation=left  Inputs=|++  SaturateOnIntegerOverflow=on
  Out1 : Outport
  wires:
  In1/1 -> Sum/1
  Sum/1 -> Integrator3/1, Integrator4/1, Out1/1
  Sum1/1 -> Sum/2
  Gain3/1 -> Gain2/1
  Gain2/1 -> Gain4/1
  Gain4/1 -> Sum1/2
  Integrator3/1 -> Integrator2/1
  Integrator4/1 -> Gain3/1
  Gain/1 -> Gain1/1
  Integrator2/1 -> Gain/1
  Gain1/1 -> Sum1/1

== system cw16/Motion Filter/High Pass Channel Angular Accelerations/transformation of scaled A/C rotations to sim Euler angle accelerations ==
  1: p (A/C) 2: q (A/C) 3: r (A/C) 4: pd (A/C) 5: qd (A/C) 6: rd (A/C) : Inport
  7: phi (Sim) 8: theta (Sim) 9: psi (Sim) 10: phid (Sim) 11: thetad (Sim) 12: psid (Sim) : Selector  InputPortWidth=21  IndexOptions=Index vector (dialog)  Indices=[7 8 9 13 14 15]  OutputSizes=1
  Mux : Mux  Inputs=3
  Mux1 : Mux  Inputs=[6 6]
  phidd : Fcn  Expr=(cos(u[7])*u[10]*tan(u[8])+sin(u[7])*(1+tan(u[8])^2)*u[11])*u[2]+(cos(u[7])*(1+tan(u[8])^2)*u[11]-sin(u[7])*u[10]*tan(u[8]))*u[3]+u[4]+sin(u[7])*tan(u[8])*u[5]+cos(u[7])*tan(u[8])*u[6]
  psidd : Fcn  Expr=((cos(u[8])*cos(u[7])*u[10]+sin(u[7])*sin(u[8])*u[11])/(cos(u[8])^2))*u[2]+((cos(u[7])*sin(u[8])*u[11]-cos(u[8])*sin(u[7])*u[10])/(cos(u[8])^2))*u[3]+((sin(u[7]))/(cos(u[8])))*u[5]+((cos(u[7]))/(cos(u[8])))*u[6]
  thetadd : Fcn  Expr=-sin(u[7])*u[10]*u[2]+cos(u[7])*u[10]*u[3]+cos(u[7])*u[5]-sin(u[7])*u[6]
  phidd thetadd psidd : Outport
  wires:
  Mux/1 -> phidd thetadd psidd/1
  thetadd/1 -> Mux/2
  phidd/1 -> Mux/1
  psidd/1 -> Mux/3
  [SimState] -> 7: phi (Sim) 8: theta (Sim) 9: psi (Sim) 10: phid (Sim) 11: thetad (Sim) 12: psid (Sim)/1
  1: p (A/C) 2: q (A/C) 3: r (A/C) 4: pd (A/C) 5: qd (A/C) 6: rd (A/C)/1 -> Mux1/1
  7: phi (Sim) 8: theta (Sim) 9: psi (Sim) 10: phid (Sim) 11: thetad (Sim) 12: psid (Sim)/1 -> Mux1/2
  Mux1/1 -> thetadd/1, phidd/1, psidd/1

== system cw16/Motion Filter/High Pass Channel Specific Forces/HP 1st order X - wb ==
  In1 : Inport
  Gain1 : Gain  Orientation=left  Gain=HPomegabx  SaturateOnIntegerOverflow=on
  Integrator2 : Integrator  Orientation=left
  Sum : Sum  Inputs=|+-  SaturateOnIntegerOverflow=on
  Out1 : Outport
  wires:
  In1/1 -> Sum/1
  Sum/1 -> Out1/1, Integrator2/1
  Integrator2/1 -> Gain1/1
  Gain1/1 -> Sum/2

== system cw16/Motion Filter/High Pass Channel Specific Forces/HP 1st order Y - wb ==
  In1 : Inport
  Gain1 : Gain  Orientation=left  Gain=HPomegaby  SaturateOnIntegerOverflow=on
  Integrator2 : Integrator  Orientation=left
  Sum : Sum  Inputs=|+-  SaturateOnIntegerOverflow=on
  Out1 : Outport
  wires:
  Gain1/1 -> Sum/2
  Integrator2/1 -> Gain1/1
  Sum/1 -> Integrator2/1, Out1/1
  In1/1 -> Sum/1

== system cw16/Motion Filter/High Pass Channel Specific Forces/HP 1st order Z - wb ==
  In1 : Inport
  Gain1 : Gain  Orientation=left  Gain=HPomegabz  SaturateOnIntegerOverflow=on
  Integrator2 : Integrator  Orientation=left
  Sum : Sum  Inputs=|+-  SaturateOnIntegerOverflow=on
  Out1 : Outport
  wires:
  In1/1 -> Sum/1
  Sum/1 -> Out1/1, Integrator2/1
  Integrator2/1 -> Gain1/1
  Gain1/1 -> Sum/2

== system cw16/Motion Filter/High Pass Channel Specific Forces/HP 2n order Z - wn ==
  In1 : Inport
  Gain : Gain  Orientation=left  Gain=HPomeganz  SaturateOnIntegerOverflow=on
  Gain1 : Gain  Orientation=left  Gain=HPomeganz  SaturateOnIntegerOverflow=on
  Gain2 : Gain  Orientation=left  Gain=HPomeganz  SaturateOnIntegerOverflow=on
  Gain3 : Gain  Orientation=left  Gain=HPzetaz  SaturateOnIntegerOverflow=on
  Gain4 : Gain  Orientation=left  Gain=2  SaturateOnIntegerOverflow=on
  Integrator2 : Integrator  Orientation=left
  Integrator3 : Integrator  Orientation=left
  Integrator4 : Integrator  Orientation=left
  Sum : Sum  Inputs=|+-  SaturateOnIntegerOverflow=on
  Sum1 : Sum  Orientation=left  Inputs=|++  SaturateOnIntegerOverflow=on
  Out1 : Outport
  wires:
  In1/1 -> Sum/1
  Sum/1 -> Integrator3/1, Integrator4/1, Out1/1
  Sum1/1 -> Sum/2
  Gain3/1 -> Gain2/1
  Gain2/1 -> Gain4/1
  Gain4/1 -> Sum1/2
  Integrator3/1 -> Integrator2/1
  Integrator4/1 -> Gain3/1
  Gain/1 -> Gain1/1
  Integrator2/1 -> Gain/1
  Gain1/1 -> Sum1/1

== system cw16/Motion Filter/High Pass Channel Specific Forces/HP 2nd order X - wn ==
  In1 : Inport
  Gain : Gain  Orientation=left  Gain=HPomeganx  SaturateOnIntegerOverflow=on
  Gain1 : Gain  Orientation=left  Gain=HPomeganx  SaturateOnIntegerOverflow=on
  Gain2 : Gain  Orientation=left  Gain=HPomeganx  SaturateOnIntegerOverflow=on
  Gain3 : Gain  Orientation=left  Gain=HPzetax  SaturateOnIntegerOverflow=on
  Gain4 : Gain  Orientation=left  Gain=2  SaturateOnIntegerOverflow=on
  Integrator2 : Integrator  Orientation=left
  Integrator3 : Integrator  Orientation=left
  Integrator4 : Integrator  Orientation=left
  Sum : Sum  Inputs=|+-  SaturateOnIntegerOverflow=on
  Sum1 : Sum  Orientation=left  Inputs=|++  SaturateOnIntegerOverflow=on
  Out1 : Outport
  wires:
  In1/1 -> Sum/1
  Sum/1 -> Integrator3/1, Integrator4/1, Out1/1
  Sum1/1 -> Sum/2
  Gain3/1 -> Gain2/1
  Gain2/1 -> Gain4/1
  Gain4/1 -> Sum1/2
  Integrator3/1 -> Integrator2/1
  Integrator4/1 -> Gain3/1
  Gain/1 -> Gain1/1
  Integrator2/1 -> Gain/1
  Gain1/1 -> Sum1/1

== system cw16/Motion Filter/High Pass Channel Specific Forces/HP 2nd order Y - wn ==
  In1 : Inport
  Gain : Gain  Orientation=left  Gain=HPomegany  SaturateOnIntegerOverflow=on
  Gain1 : Gain  Orientation=left  Gain=HPomegany  SaturateOnIntegerOverflow=on
  Gain2 : Gain  Orientation=left  Gain=HPomegany  SaturateOnIntegerOverflow=on
  Gain3 : Gain  Orientation=left  Gain=HPzetay  SaturateOnIntegerOverflow=on
  Gain4 : Gain  Orientation=left  Gain=2  SaturateOnIntegerOverflow=on
  Integrator2 : Integrator  Orientation=left
  Integrator3 : Integrator  Orientation=left
  Integrator4 : Integrator  Orientation=left
  Sum : Sum  Inputs=|+-  SaturateOnIntegerOverflow=on
  Sum1 : Sum  Orientation=left  Inputs=|++  SaturateOnIntegerOverflow=on
  Out1 : Outport
  wires:
  In1/1 -> Sum/1
  Sum/1 -> Integrator3/1, Integrator4/1, Out1/1
  Sum1/1 -> Sum/2
  Gain3/1 -> Gain2/1
  Gain2/1 -> Gain4/1
  Gain4/1 -> Sum1/2
  Integrator3/1 -> Integrator2/1
  Integrator4/1 -> Gain3/1
  Gain/1 -> Gain1/1
  Integrator2/1 -> Gain/1
  Gain1/1 -> Sum1/1

== system cw16/Motion Filter/High Pass Channel Specific Forces/transformation from body to inertial frame of reference ==
  note: rotation matrix L_IS, from equation 2.10 in the UTIAS document
  fxS fyS fzS : Inport
  Fcn1 : Fcn  Expr=u(1)*cos(u(5))*sin(u(6)) + u(2)*(sin(u(4))*sin(u(5))*sin(u(6))+cos(u(4))*cos(u(6))) + u(3)*(cos(u(4))*sin(u(5))*sin(u(6))-sin(u(4))*cos(u(6)))
  Fcn2 : Fcn  Expr=-u(1)*sin(u(5)) + u(2)*sin(u(4))*cos(u(5)) + u(3)*cos(u(4))*cos(u(5))
  Fcn9 : Fcn  Expr=u(1)*cos(u(5))*cos(u(6)) + u(2)*(sin(u(4))*sin(u(5))*cos(u(6))-cos(u(4))*sin(u(6))) + u(3)*(cos(u(4))*sin(u(5))*cos(u(6))+sin(u(4))*sin(u(6)))
  Mux : Mux  Inputs=3
  Mux1 : Mux  Inputs=[3 3]
  phi theta psi : Selector  InputPortWidth=21  IndexOptions=Index vector (dialog)  Indices=[7 8 9]  OutputSizes=1
  fxI fyI fzI : Outport
  wires:
  Fcn1/1 -> Mux/2
  Mux/1 -> fxI fyI fzI/1
  Fcn9/1 -> Mux/1
  Fcn2/1 -> Mux/3
  fxS fyS fzS/1 -> Mux1/1
  Mux1/1 -> Fcn9/1, Fcn1/1, Fcn2/1
  [SimState] -> phi theta psi/1
  phi theta psi/1 -> Mux1/2

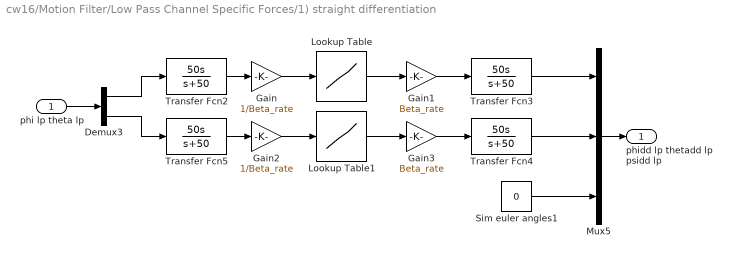
== system cw16/Motion Filter/Low Pass Channel Specific Forces/1) straight differentiation ==
  phi lp theta lp : Inport
  Demux3 : Demux  Outputs=2
  Gain : Gain  Gain=1/Beta_rate
  Gain1 : Gain  Gain=Beta_rate
  Gain2 : Gain  Gain=1/Beta_rate
  Gain3 : Gain  Gain=Beta_rate
  Lookup Table : Lookup_n-D  NumberOfTableDimensions=1  BreakpointsForDimension1=[-5:0.05:5]  Table=tanh([-5:0.05:5])  ExtrapMethod=None - Clip
  Lookup Table1 : Lookup_n-D  NumberOfTableDimensions=1  BreakpointsForDimension1=[-5:0.05:5]  Table=tanh([-5:0.05:5])  ExtrapMethod=None - Clip
  Mux5 : Mux  Inputs=3
  Sim euler angles1 : Constant  Value=0
  Transfer Fcn{2..5} (4 alike) : TransferFcn  Numerator=[50 0]  Denominator=[1 50]
  phidd lp thetadd lp psidd lp : Outport
  wires:
  Demux3/1 -> Transfer Fcn2/1
  Sim euler angles1/1 -> Mux5/3
  Transfer Fcn3/1 -> Mux5/1
  Demux3/2 -> Transfer Fcn5/1
  Transfer Fcn4/1 -> Mux5/2
  phi lp theta lp/1 -> Demux3/1
  Mux5/1 -> phidd lp thetadd lp psidd lp/1
  Gain/1 -> Lookup Table/1
  Lookup Table/1 -> Gain1/1
  Gain2/1 -> Lookup Table1/1
  Lookup Table1/1 -> Gain3/1
  Transfer Fcn2/1 -> Gain/1
  Transfer Fcn5/1 -> Gain2/1
  Gain1/1 -> Transfer Fcn3/1
  Gain3/1 -> Transfer Fcn4/1

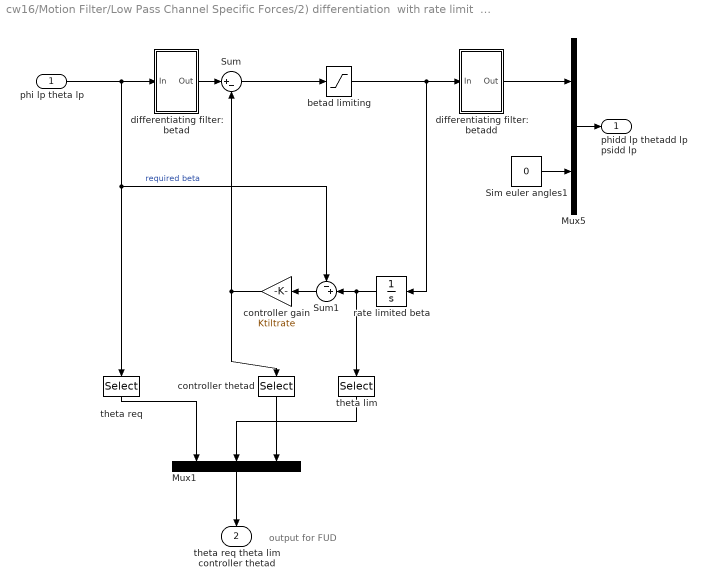
== system cw16/Motion Filter/Low Pass Channel Specific Forces/2) differentiation  with rate limit  compensation ==
  note: output for FUD
  phi lp theta lp : Inport
  Mux1 : Mux  Orientation=down  Inputs=3
  Mux5 : Mux  Inputs=[2 1]
  Sim euler angles1 : Constant  Value=0
  Sum : Sum  Inputs=|+-  SaturateOnIntegerOverflow=on
  Sum1 : Sum  Orientation=left  Inputs=-+|  SaturateOnIntegerOverflow=on
  betad limiting : Saturate  UpperLimit=Beta_rate  LowerLimit=-Beta_rate
  controller gain : Gain  Orientation=left  Gain=Ktiltrate  SaturateOnIntegerOverflow=on
  controller thetad : Selector  Orientation=down  InputPortWidth=2  IndexOptions=Index vector (dialog)  Indices=[2]  OutputSizes=1
  differentiating filter: betad : Subsystem
  differentiating filter: betadd : Subsystem
  rate limited beta : Integrator  Orientation=left
  theta lim : Selector  Orientation=down  InputPortWidth=2  IndexOptions=Index vector (dialog)  Indices=[2]  OutputSizes=1
  theta req : Selector  Orientation=down  InputPortWidth=2  IndexOptions=Index vector (dialog)  Indices=[2]  OutputSizes=1
  phidd lp thetadd lp psidd lp : Outport
  theta req theta lim controller thetad : Outport  Orientation=down  Port=2
  wires:
  Mux5/1 -> phidd lp thetadd lp psidd lp/1
  phi lp theta lp/1 -> differentiating filter: betad/1(In), Sum1/1, theta req/1  "required beta"
  differentiating filter: betadd/1(Out) -> Mux5/1
  Sim euler angles1/1 -> Mux5/2
  betad limiting/1 -> differentiating filter: betadd/1(In), rate limited beta/1
  differentiating filter: betad/1(Out) -> Sum/1
  Sum/1 -> betad limiting/1
  controller gain/1 -> Sum/2, controller thetad/1
  rate limited beta/1 -> theta lim/1, Sum1/2
  Sum1/1 -> controller gain/1
  theta req/1 -> Mux1/1
  theta lim/1 -> Mux1/2
  Mux1/1 -> theta req theta lim controller thetad/1
  controller thetad/1 -> Mux1/3

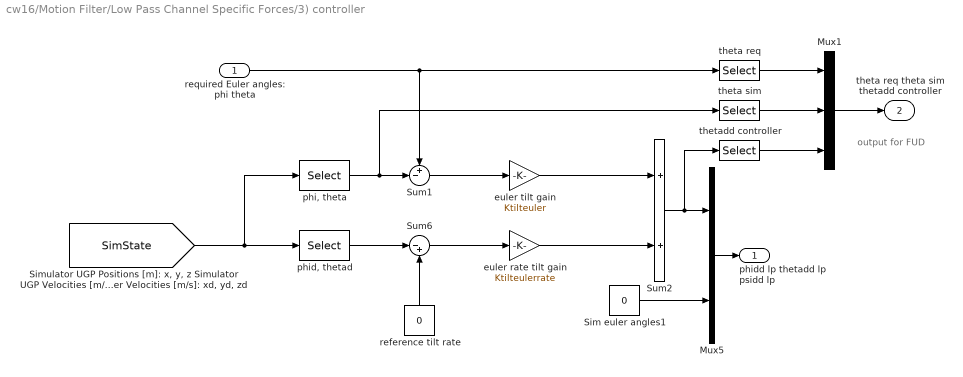
== system cw16/Motion Filter/Low Pass Channel Specific Forces/3) controller ==
  note: output for FUD
  required Euler angles: phi theta : Inport
  Mux1 : Mux  Inputs=3
  Mux5 : Mux  Inputs=2
  Sim euler angles1 : Constant  Value=0
  Sum1 : Sum  Inputs=+-|  SaturateOnIntegerOverflow=on  InputSameDT=on
  Sum2 : Sum  SaturateOnIntegerOverflow=on  InputSameDT=on
  Sum6 : Sum  Inputs=|-+  SaturateOnIntegerOverflow=on  InputSameDT=on
  euler rate tilt gain : Gain  Gain=Ktilteulerrate  SaturateOnIntegerOverflow=on
  euler tilt gain : Gain  Gain=Ktilteuler  SaturateOnIntegerOverflow=on
  "phi, theta" : Selector  InputPortWidth=21  IndexOptions=Index vector (dialog)  Indices=[7 8]  OutputSizes=1
  "phid, thetad" : Selector  InputPortWidth=21  IndexOptions=Index vector (dialog)  Indices=[13 14]  OutputSizes=1
  reference tilt rate : Constant  Orientation=up  Value=0
  theta req : Selector  InputPortWidth=2  IndexOptions=Index vector (dialog)  Indices=[2]  OutputSizes=1
  theta sim : Selector  InputPortWidth=2  IndexOptions=Index vector (dialog)  Indices=[2]  OutputSizes=1
  thetadd controller : Selector  InputPortWidth=2  IndexOptions=Index vector (dialog)  Indices=[2]  OutputSizes=1
  phidd lp thetadd lp psidd lp : Outport
  "theta req theta sim thetadd controller " : Outport  Port=2
  wires:
  Sim euler angles1/1 -> Mux5/2
  Mux5/1 -> phidd lp thetadd lp psidd lp/1
  Sum1/1 -> euler tilt gain/1
  "phi, theta"/1 -> Sum1/2, theta sim/1
  required Euler angles: phi theta/1 -> Sum1/1, theta req/1
  euler tilt gain/1 -> Sum2/1
  Sum6/1 -> euler rate tilt gain/1
  "phid, thetad"/1 -> Sum6/1
  reference tilt rate/1 -> Sum6/2
  euler rate tilt gain/1 -> Sum2/2
  Sum2/1 -> Mux5/1, thetadd controller/1
  theta req/1 -> Mux1/1
  Mux1/1 -> "theta req theta sim thetadd controller "/1
  thetadd controller/1 -> Mux1/3
  theta sim/1 -> Mux1/2
  [SimState] -> "phi, theta"/1, "phid, thetad"/1

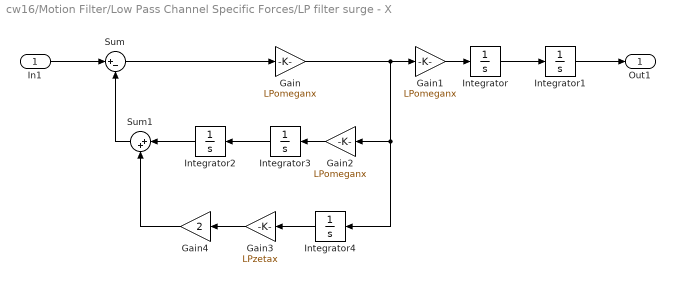
== system cw16/Motion Filter/Low Pass Channel Specific Forces/LP filter surge - X  ==
  In1 : Inport
  Gain : Gain  Gain=LPomeganx  SaturateOnIntegerOverflow=on
  Gain1 : Gain  Gain=LPomeganx  SaturateOnIntegerOverflow=on
  Gain2 : Gain  Orientation=left  Gain=LPomeganx  SaturateOnIntegerOverflow=on
  Gain3 : Gain  Orientation=left  Gain=LPzetax  SaturateOnIntegerOverflow=on
  Gain4 : Gain  Orientation=left  Gain=2  SaturateOnIntegerOverflow=on
  Integrator : Integrator
  Integrator1 : Integrator
  Integrator2 : Integrator  Orientation=left
  Integrator3 : Integrator  Orientation=left
  Integrator4 : Integrator  Orientation=left
  Sum : Sum  Inputs=|+-  SaturateOnIntegerOverflow=on
  Sum1 : Sum  Orientation=left  Inputs=|++  SaturateOnIntegerOverflow=on
  Out1 : Outport
  wires:
  In1/1 -> Sum/1
  Sum/1 -> Gain/1
  Gain/1 -> Integrator4/1, Gain2/1, Gain1/1
  Integrator/1 -> Integrator1/1
  Integrator1/1 -> Out1/1
  Sum1/1 -> Sum/2
  Integrator2/1 -> Sum1/1
  Gain3/1 -> Gain4/1
  Gain4/1 -> Sum1/2
  Integrator3/1 -> Integrator2/1
  Integrator4/1 -> Gain3/1
  Gain1/1 -> Integrator/1
  Gain2/1 -> Integrator3/1

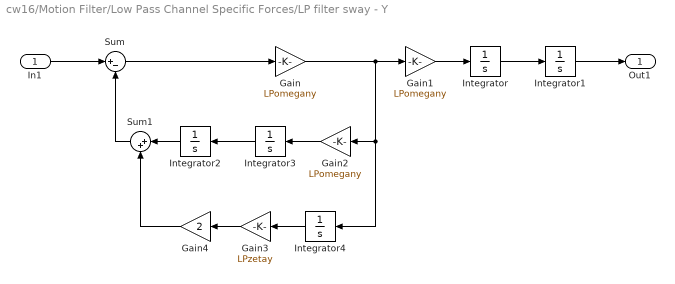
== system cw16/Motion Filter/Low Pass Channel Specific Forces/LP filter sway - Y  ==
  In1 : Inport
  Gain : Gain  Gain=LPomegany  SaturateOnIntegerOverflow=on
  Gain1 : Gain  Gain=LPomegany  SaturateOnIntegerOverflow=on
  Gain2 : Gain  Orientation=left  Gain=LPomegany  SaturateOnIntegerOverflow=on
  Gain3 : Gain  Orientation=left  Gain=LPzetay  SaturateOnIntegerOverflow=on
  Gain4 : Gain  Orientation=left  Gain=2  SaturateOnIntegerOverflow=on
  Integrator : Integrator
  Integrator1 : Integrator
  Integrator2 : Integrator  Orientation=left
  Integrator3 : Integrator  Orientation=left
  Integrator4 : Integrator  Orientation=left
  Sum : Sum  Inputs=|+-  SaturateOnIntegerOverflow=on
  Sum1 : Sum  Orientation=left  Inputs=|++  SaturateOnIntegerOverflow=on
  Out1 : Outport
  wires:
  In1/1 -> Sum/1
  Sum/1 -> Gain/1
  Gain/1 -> Integrator4/1, Gain2/1, Gain1/1
  Integrator/1 -> Integrator1/1
  Integrator1/1 -> Out1/1
  Sum1/1 -> Sum/2
  Integrator2/1 -> Sum1/1
  Gain3/1 -> Gain4/1
  Gain4/1 -> Sum1/2
  Integrator3/1 -> Integrator2/1
  Integrator4/1 -> Gain3/1
  Gain1/1 -> Integrator/1
  Gain2/1 -> Integrator3/1

== system cw16/Motion Filter/Low Pass Channel Specific Forces/2) differentiation  with rate limit  compensation/differentiating filter: betad ==
  In : Inport
  Demux3 : Demux  Outputs=2
  Mux : Mux  Inputs=2
  Transfer Fcn2 : TransferFcn  Numerator=[12.5 0]  Denominator=[1 12.5]
  Transfer Fcn5 : TransferFcn  Numerator=[12.5 0]  Denominator=[1 12.5]
  Out : Outport
  wires:
  Demux3/2 -> Transfer Fcn5/1
  Demux3/1 -> Transfer Fcn2/1
  Transfer Fcn2/1 -> Mux/1
  In/1 -> Demux3/1
  Transfer Fcn5/1 -> Mux/2
  Mux/1 -> Out/1

== system cw16/Motion Filter/Low Pass Channel Specific Forces/2) differentiation  with rate limit  compensation/differentiating filter: betadd ==
  In : Inport
  Demux3 : Demux  Outputs=2
  Mux : Mux  Inputs=2
  Transfer Fcn2 : TransferFcn  Numerator=[12.5 0]  Denominator=[1 12.5]
  Transfer Fcn5 : TransferFcn  Numerator=[12.5 0]  Denominator=[1 12.5]
  Out : Outport
  wires:
  Demux3/2 -> Transfer Fcn5/1
  Demux3/1 -> Transfer Fcn2/1
  Transfer Fcn2/1 -> Mux/1
  In/1 -> Demux3/1
  Transfer Fcn5/1 -> Mux/2
  Mux/1 -> Out/1
